simulink model "nivel"  (R2020a)
settings: Solver=VariableStepAuto  StartTime=0.0  StopTime=10000  RelTol=1e-3
settings Model: Creator=gabriel  LastModifiedBy=gabriel

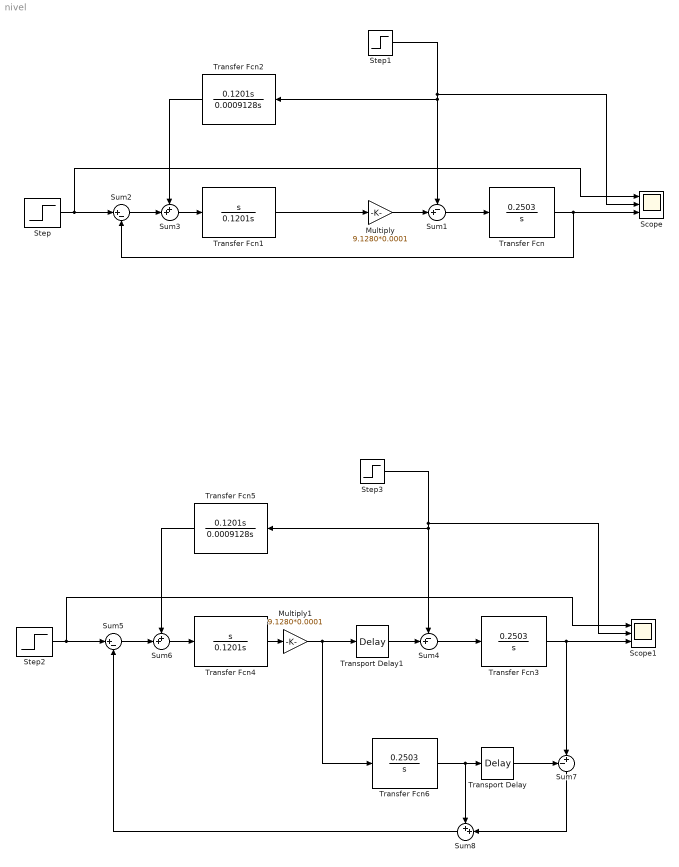
== system nivel ==
  Multiply : Gain  Gain=9.1280*0.0001
  Multiply1 : Gain  Gain=9.1280*0.0001
  Scope : Scope  NumInputPorts=3
  Scope1 : Scope  NumInputPorts=3
  Step : Step  Time=100  SampleTime=0
  Step1 : Step  Time=5000  SampleTime=0
  Step2 : Step  Time=100  SampleTime=0
  Step3 : Step  Time=5000  SampleTime=0
  Sum1 : Sum  Inputs=-+|
  Sum2 : Sum  Inputs=|+-
  Sum3 : Sum  Inputs=++|
  Sum4 : Sum  Inputs=-+|
  Sum5 : Sum  Inputs=|+-
  Sum6 : Sum  Inputs=++|
  Sum7 : Sum  Inputs=-+|
  Sum8 : Sum  Inputs=++|
  Transfer Fcn : TransferFcn  Numerator=[0.2503]  Denominator=[1 0]
  Transfer Fcn1 : TransferFcn  Numerator=[1 0]  Denominator=[0.1201 0]
  Transfer Fcn2 : TransferFcn  Numerator="[0.1201  0]"  Denominator=[0.0009128 0]
  Transfer Fcn3 : TransferFcn  Numerator=[0.2503]  Denominator=[1 0]
  Transfer Fcn4 : TransferFcn  Numerator=[1 0]  Denominator=[0.1201 0]
  Transfer Fcn5 : TransferFcn  Numerator="[0.1201  0]"  Denominator=[0.0009128 0]
  Transfer Fcn6 : TransferFcn  Numerator=[0.2503]  Denominator=[1 0]
  Transport Delay : TransportDelay
  Transport Delay1 : TransportDelay
  wires:
  Multiply/1 -> Sum1/2
  Sum1/1 -> Transfer Fcn/1
  Transfer Fcn/1 -> Sum2/2, Scope/3
  Transfer Fcn1/1 -> Multiply/1
  Step/1 -> Scope/1, Sum2/1
  Step1/1 -> Scope/2, Sum1/1, Transfer Fcn2/1
  Sum2/1 -> Sum3/2
  Sum3/1 -> Transfer Fcn1/1
  Transfer Fcn2/1 -> Sum3/1
  Step3/1 -> Scope1/2, Sum4/1, Transfer Fcn5/1
  Sum5/1 -> Sum6/2
  Multiply1/1 -> Transfer Fcn6/1, Transport Delay1/1
  Step2/1 -> Scope1/1, Sum5/1
  Transfer Fcn5/1 -> Sum6/1
  Sum6/1 -> Transfer Fcn4/1
  Transfer Fcn4/1 -> Multiply1/1
  Transfer Fcn3/1 -> Sum7/2, Scope1/3
  Sum4/1 -> Transfer Fcn3/1
  Transport Delay/1 -> Sum7/1
  Transfer Fcn6/1 -> Sum8/1, Transport Delay/1
  Transport Delay1/1 -> Sum4/2
  Sum7/1 -> Sum8/2
  Sum8/1 -> Sum5/2
